simulink model "control_PID"  (R2022b)
settings: Solver=VariableStepAuto  StartTime=0.0  StopTime=200  RelTol=1e-3
libraries: fuzblock x3
settings Model: Creator=Coordinación  LastModifiedBy=sophy

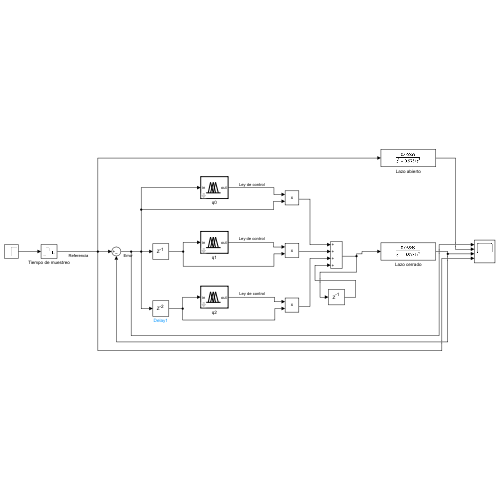
[thumbnail: Simulink's stored preview of the top-level diagram]
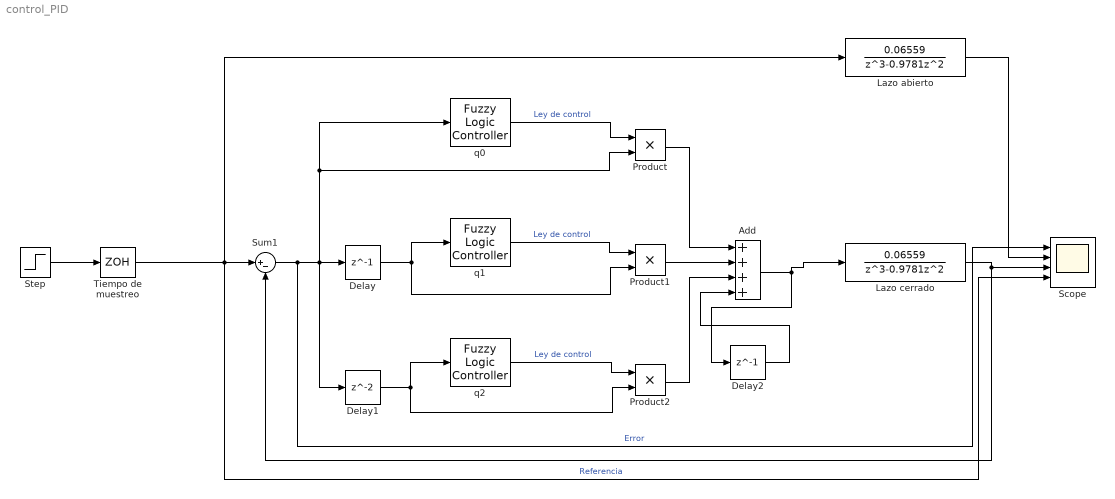
== system control_PID ==
  Add : Sum  Inputs=++++
  Delay : Delay  DelayLength=1
  Delay1 : Delay
  Delay2 : Delay  DelayLength=1
  Lazo abierto : DiscreteTransferFcn  Numerator=[0.06559]  Denominator=[1 -0.9781 0 0]
  Lazo cerrado : DiscreteTransferFcn  Numerator=[0.06559]  Denominator=[1 -0.9781 0 0]
  Product : Product
  Product1 : Product
  Product2 : Product
  Scope : Scope  NumInputPorts=4
  Step : Step  Time=0  After=10  SampleTime=0
  Sum1 : Sum  Inputs=|+-
  Tiempo de muestreo : ZeroOrderHold  SampleTime=1.05
  q0 : fuzblock/Fuzzy Logic  Controller  FIS=q0_PID  OutputSampleNumber=101  DataType=double  FuzzifiedInputs=off  RuleFiringStrengths=off  RuleOutputs=off  AggregatedOutputs=off  SimulateUsing=Interpreted execution  OutOfRangeInputValueMessage=warning  NoRuleFiredMessage=warning  EmptyOutputFuzzySetMessage=warning
  q1 : fuzblock/Fuzzy Logic  Controller  FIS=q1_PID  OutputSampleNumber=101  DataType=double  FuzzifiedInputs=off  RuleFiringStrengths=off  RuleOutputs=off  AggregatedOutputs=off  SimulateUsing=Interpreted execution  OutOfRangeInputValueMessage=warning  NoRuleFiredMessage=warning  EmptyOutputFuzzySetMessage=warning
  q2 : fuzblock/Fuzzy Logic  Controller  FIS=q2_PID  OutputSampleNumber=101  DataType=double  FuzzifiedInputs=off  RuleFiringStrengths=off  RuleOutputs=off  AggregatedOutputs=off  SimulateUsing=Interpreted execution  OutOfRangeInputValueMessage=warning  NoRuleFiredMessage=warning  EmptyOutputFuzzySetMessage=warning
  wires:
  Sum1/1 -> Scope/1, Delay/1, q0/1, Product/2, Delay1/1  "Error"
  q0/1 -> Product/1  "Ley de control"
  Delay/1 -> Product1/2, q1/1
  q1/1 -> Product1/1  "Ley de control"
  Product/1 -> Add/1
  Product1/1 -> Add/2
  Add/1 -> Lazo cerrado/1, Delay2/1
  Lazo cerrado/1 -> Scope/3, Sum1/2
  Lazo abierto/1 -> Scope/2
  Delay1/1 -> q2/1, Product2/2
  q2/1 -> Product2/1  "Ley de control"
  Product2/1 -> Add/3
  Tiempo de muestreo/1 -> Scope/4, Lazo abierto/1, Sum1/1  "Referencia"
  Step/1 -> Tiempo de muestreo/1
  Delay2/1 -> Add/4
